simulink model "mvdc_exactlin_feedback"  (R2018b)
settings: configuration reference "Active" (kept outside this file)
undefined symbols (not defined in the file): drag_coefficient, l_front_m, l_rear_m, P_VDC_EL_alphaMax_rad, P_VDC_EL_axMaxFB_mps2, P_VDC_EL_c_1prad, P_VDC_EL_c_F_N, P_VDC_EL_c_R_N, P_VDC_EL_FxStandstill_N, P_VDC_EL_LatControl_w_0, P_VDC_EL_vFullControl_mps, P_VDC_LatControl_D, P_VDC_LongControl_Kp, P_VDC_MinVelSlipCalc_mps, roh_air, vehiclemass_kg
libraries: simulink x2
settings Model: DataDictionary=mvdc_exactlin_feedback.sldd  Creator=wischnewski  LastModifiedBy=ge34qer

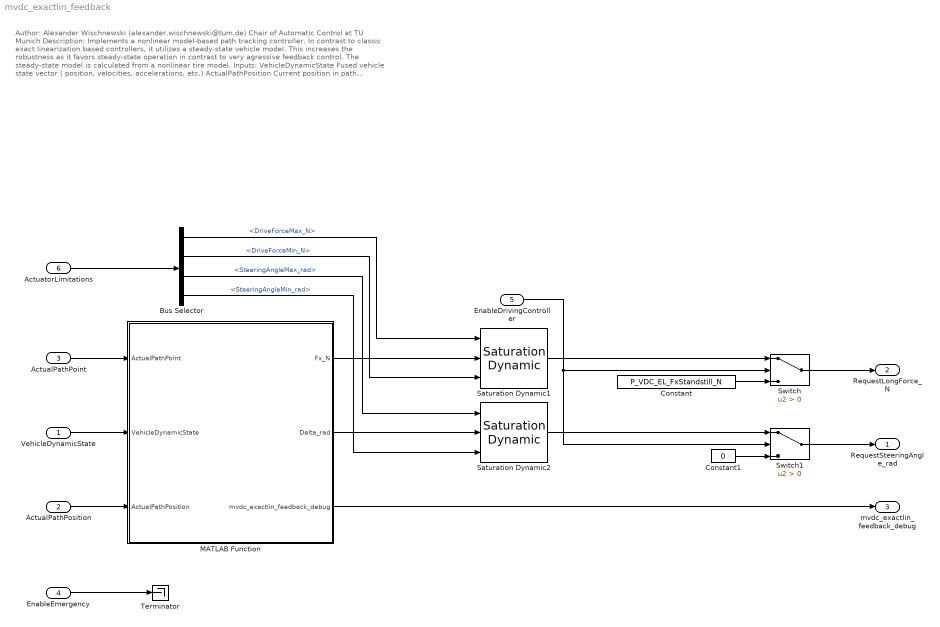
== system mvdc_exactlin_feedback ==
  note: Author: Alexander Wischnewski (alexander.wischnewski@tum.de)
      | Chair of Automatic Control at TU Munich
      |
      | Description: Implements a nonlinear model-based path tracking controller. In contrast to classic exact
      | linearization based controllers, it utilizes a steady-state vehicle model. This increases the robustness
      | as it favors steady-state operation in contrast to very agressive feedback control. The steady-state model is
      | calculated from a nonlinear tire model.
      |
      | Inputs:
      | VehicleDynamicState Fused vehicle state vector ( position, velocities, accelerations, etc.)
      | ActualPathPosition Current position in path coordinates
      | ActualPathPoint Current point matched on the target trajectory
      | EnableEmergency Signalize controller that an emergency has been triggered
      | EnableDrivingController Signalize controller that it is allowed to drive now
      | ActuatorLimitations Hardware limitations of the actuators
      |
      | Outputs:
      | RequestSteeringAngle_rad Requested steering angle at the wheel
      | RequestLongForce_N Requested long traction force
  VehicleDynamicState : Inport  OutDataTypeStr=Bus: VehicleDynamicState
  ActualPathPosition : Inport  Port=2  OutDataTypeStr=Bus: PathPos  PortDimensions=1  BusOutputAsStruct=on
  ActualPathPoint : Inport  Port=3  OutDataTypeStr=Bus: PathPoint  PortDimensions=1  BusOutputAsStruct=on
  EnableEmergency : Inport  Port=4  OutDataTypeStr=boolean
  EnableDrivingController : Inport  Port=5  OutDataTypeStr=boolean  PortDimensions=1  BusOutputAsStruct=on
  ActuatorLimitations : Inport  Port=6  OutDataTypeStr=Bus: ActuatorLimitations  BusOutputAsStruct=on
  Bus Selector : BusSelector  OutputSignals=DriveForceMax_N,DriveForceMin_N,SteeringAngleMax_rad,SteeringAngleMin_rad
  Constant : Constant  Value=P_VDC_EL_FxStandstill_N
  Constant1 : Constant  Value=0
  MATLAB Function : MATLAB Function  TreatAsAtomicUnit=on
  Saturation Dynamic1 : simulink/Discontinuities/Saturation Dynamic  OutMin=[]  OutMax=[]  OutDataTypeStr=Inherit: Same as second input  OutDataType=fixdt(1, 16)  OutScaling=2^-10  DoSatur=off
  Saturation Dynamic2 : simulink/Discontinuities/Saturation Dynamic  OutMin=[]  OutMax=[]  OutDataTypeStr=Inherit: Same as second input  OutDataType=fixdt(1, 16)  OutScaling=2^-10  DoSatur=off
  Switch : Switch  Criteria=u2 > Threshold
  Switch1 : Switch  Criteria=u2 > Threshold
  Terminator : Terminator
  RequestSteeringAngle_rad : Outport
  RequestLongForce_N : Outport  Port=2
  mvdc_exactlin_feedback_debug : Outport  Port=3  OutDataTypeStr=Bus: mvdc_exactlin_feedback_debug
  wires:
  VehicleDynamicState/1 -> MATLAB Function/2(VehicleDynamicState)
  ActualPathPoint/1 -> MATLAB Function/1(ActualPathPoint)
  ActualPathPosition/1 -> MATLAB Function/3(ActualPathPosition)
  Saturation Dynamic1/1 -> Switch/1
  Saturation Dynamic2/1 -> Switch1/1
  EnableDrivingController/1 -> Switch/2, Switch1/2
  Constant/1 -> Switch/3
  Constant1/1 -> Switch1/3
  Switch/1 -> RequestLongForce_N/1
  Switch1/1 -> RequestSteeringAngle_rad/1
  MATLAB Function/3(mvdc_exactlin_feedback_debug) -> mvdc_exactlin_feedback_debug/1
  EnableEmergency/1 -> Terminator/1
  MATLAB Function/2(Delta_rad) -> Saturation Dynamic2/2
  MATLAB Function/1(Fx_N) -> Saturation Dynamic1/2
  ActuatorLimitations/1 -> Bus Selector/1
  Bus Selector/4 -> Saturation Dynamic2/3  "<SteeringAngleMin_rad>"
  Bus Selector/3 -> Saturation Dynamic2/1  "<SteeringAngleMax_rad>"
  Bus Selector/2 -> Saturation Dynamic1/3  "<DriveForceMin_N>"
  Bus Selector/1 -> Saturation Dynamic1/1  "<DriveForceMax_N>"

== matlab function mvdc_exactlin_feedback/MATLAB Function ==
  data: ActualPathPoint input Bus: PathPoint; Fx_N output; VehicleDynamicState input Bus: VehicleDynamicState; ActualPathPosition input Bus: PathPos; Delta_rad output; mvdc_exactlin_feedback_debug output Bus: mvdc_exactlin_feedback_debug; vehiclemass_kg parameter; roh_air parameter; drag_coefficient parameter; l_front_m parameter; l_rear_m parameter; P_VDC_MinVelSlipCalc_mps parameter; P_VDC_EL_axMaxFB_mps2 parameter; P_VDC_EL_c_F_N parameter; P_VDC_EL_c_R_N parameter; P_VDC_EL_c_1prad parameter; P_VDC_EL_alphaMax_rad parameter; P_VDC_EL_vFullControl_mps parameter; P_VDC_EL_LatControl_w_0 parameter; P_VDC_LatControl_D parameter; P_VDC_LongControl_Kp parameter
function [Fx_N, Delta_rad, mvdc_exactlin_feedback_debug] = exactlin_feedback(ActualPathPoint, VehicleDynamicState, ActualPathPosition, vehiclemass_kg, roh_air, drag_coefficient, l_front_m, l_rear_m, P_VDC_MinVelSlipCalc_mps,...
    P_VDC_EL_axMaxFB_mps2, P_VDC_EL_c_F_N, P_VDC_EL_c_R_N, P_VDC_EL_c_1prad, P_VDC_EL_alphaMax_rad, P_VDC_EL_vFullControl_mps, P_VDC_EL_LatControl_w_0, P_VDC_LatControl_D, P_VDC_LongControl_Kp)

[Fx_N, Delta_rad, mvdc_exactlin_feedback_debug] = exactlin_feedback(ActualPathPoint, VehicleDynamicState, ActualPathPosition, vehiclemass_kg, roh_air, drag_coefficient, l_front_m, l_rear_m, P_VDC_MinVelSlipCalc_mps,...
    P_VDC_EL_axMaxFB_mps2, P_VDC_EL_c_F_N, P_VDC_EL_c_R_N, P_VDC_EL_c_1prad, P_VDC_EL_alphaMax_rad, P_VDC_EL_vFullControl_mps, P_VDC_EL_LatControl_w_0, P_VDC_LatControl_D, P_VDC_LongControl_Kp);
